simulink model "Cart_pole_adaptive_simulation"  (R2025b)
settings: Solver=ode4  StartTime=0.0  StopTime=10  FixedStep=0.025  RelTol=1e-3
values from neighbouring files (symbols this model uses):
  m = 0.7    [cart_pole_model.m]    (also in cart_pole_model_2.m = SX.sym('m'))
  N = 10    [cart_pole_mhe.m]    (also in cart_pole_ocp.m = 40; test.m = round(T_sim/dt))
  s = sin(theta)    [cart_pole_adaptive_model.m]    (also in cart_pole_model.m; cart_pole_model_2.m; test.m = sin(th))
  T = 1    [cart_pole_ocp.m]
undefined symbols (not defined in the file or in its folder): X, Y, Z
libraries: sm_lib x14, nesl_utility x7
settings Model: Creator=oj  LastModifiedBy=angel
settings SolverCC: AlgebraicLoopSolver=TrustRegion
settings DataIOCC: SaveFormat=StructureWithTime
settings OptimizationCC: LifeSpan=inf
settings DebuggingCC: UnconnectedInputMsg=warning  UnconnectedOutputMsg=warning  UnconnectedLineMsg=warning  SFExecutionAtInitializationDiag=none  ArithmeticOperatorsInVariantConditions=warning
settings HardwareCC: ProdBitPerSizeT=32.0  ProdBitPerPtrDiffT=32.0  ProdWordSize=32.0  ProdHWDeviceType=Specified
settings ModelReferenceCC: EnableRefExpFcnMdlSchedulingChecks=on
settings SFSimCC: CustomCodeUndefinedFunction=UseInterfaceOnly
settings RTWCC: GPUComputeCapability=3.5
settings CodeAppCC: StateflowObjectComments=on
settings ExplorerConfigSet: InternalSimMechanicsExplorerSettings=|
  | <ExplorerConfiguration>
  | 
  |   <canonicalview>default</canonicalview>
  | 
  |   <TilePanel>
  |     <TileInfo>
  |       <Tiles Columns="1" Count="1" Height="858" Rows="1" Width="1140">
  |         <Row Weight="1"/>
  |         <Column Weight="1"/>
  |         <Tile Height="1" Width="1" X="0" Y="0"/>
  |       </Tiles>
  |     </TileInfo>
  |     <SceneInfo>
  |       <SceneViewer>
  |         <IsThisViewStd>
  |           <IsStandardView>off</IsStandardView>
  |           <StandardViewName>Front</StandardViewName>
  |         </IsThisViewStd>
  |         <BGColor>
  |           <R>1</R>
  |           <G>1</G>
  |           <B>1</B>
  |           <A>1</A>
  |         </BGColor>
  |         <Camera>
  |           <DoPerspective>off</DoPerspective>
  |           <Position>
  |             <X>0.79287567589367203</X>
  |             <Y>-2.8977650595772118</Y>
  |             <Z>0.43288588007438944</Z>
  |           </Position>
  |           <Center>
  |             <X>0.09273481289714941</X>
  |             <Y>-0.01114024585481534</Y>
  |             <Z>-0.08401232882620252</Z>
  |           </Center>
  |           <Up>
  |             <X>-0.027084665030150518</X>
  |             <Y>0.16982947078524466</Y>
  |             <Z>0.98510119874711777</Z>
  |           </Up>
  |           <XLim>0.48380424524844262</XLim>
  |           <YLim>0.48380424524844262</YLim>
  |           <ViewLimDist>0.01</ViewLimDist>
  |         </Camera>
  |       </SceneViewer>
  |     </SceneInfo>
  |   </TilePanel>
  | 
  |   <MechEditorPanel>
  |     <GfxPanelCameraMap/>
  |     <Cameras/>
  |     <VideoCreator>
  |       <IncludeTiles>All</IncludeTiles>
  |       <IncludeTime>on</IncludeTime>
  |       <IncludeWorldFrame>off</IncludeWorldFrame>
  |       <PlaybackSpeedRatio>1</PlaybackSpeedRatio>
  |       <FrameRate>30</FrameRate>
  |       <FrameSize>auto</FrameSize>
  |       <VideoFormat>UncompressedAVI</VideoFormat>
  |     </VideoCreator>
  |   </MechEditorPanel>
  | 
  |   <PlaybackSettings>
  |     <PlaybackSpeedFactor>1</PlaybackSpeedFactor>
  |   </PlaybackSettings>
  | 
  | </ExplorerConfiguration>

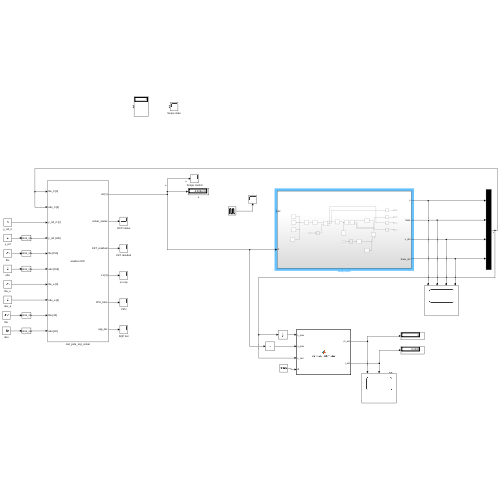
[thumbnail: Simulink's stored preview of the top-level diagram]
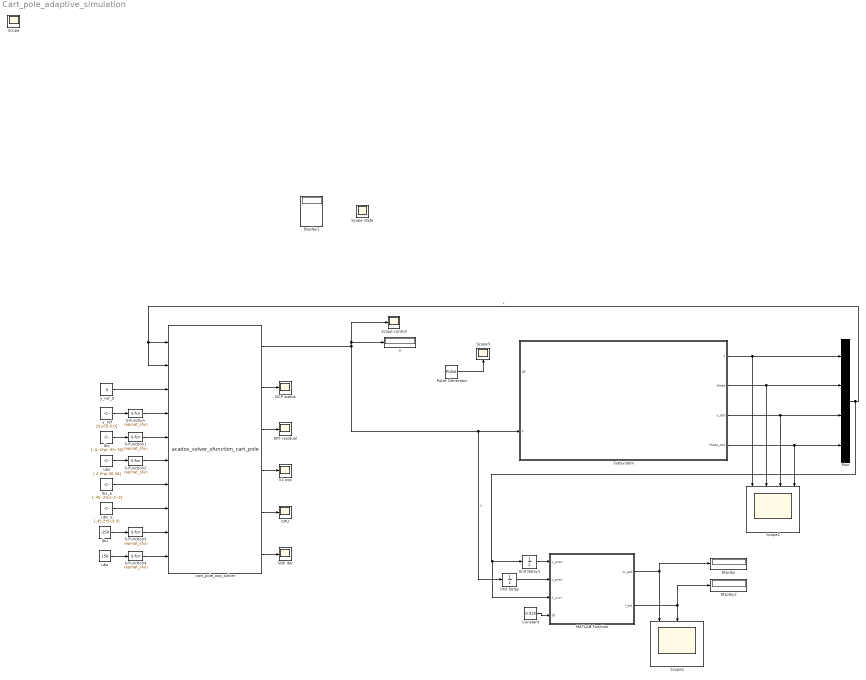
== system Cart_pole_adaptive_simulation ==
  CPU : Scope
      settings: Description=status  DataLoggingVariableName=ScopeData3
  Constant : Constant  Value=0.025
  Display : Display
  Display1 : Display
  Display2 : Display
  KKT residual : Scope
      settings: Description=status  ActiveDisplayYMinimum=-3E-6  ActiveDisplayYMaximum=3.1E-5  DataLoggingVariableName=ScopeData4
  MATLAB Function : MATLAB Function  TreatAsAtomicUnit=on
  Mux : Mux
  OCP status : Scope
      settings: Description=status  ActiveDisplayYMinimum=-4.610104567980212  ActiveDisplayYMaximum=5.6802344204737647
  Pulse Generator : DiscretePulseGenerator  PulseType=Time based  Period=10  PulseWidth=10  PhaseDelay=3
  S-Function : S-Function  FunctionName=repmat_sfun  Parameters=N/T-1  SFunctionDeploymentMode=off  EnableBusSupport=off
  S-Function1 : S-Function  FunctionName=repmat_sfun  Parameters=N/T-1  SFunctionDeploymentMode=off  EnableBusSupport=off
  S-Function2 : S-Function  FunctionName=repmat_sfun  Parameters=N/T-1  SFunctionDeploymentMode=off  EnableBusSupport=off
  S-Function3 : S-Function  FunctionName=repmat_sfun  Parameters=N  SFunctionDeploymentMode=off  EnableBusSupport=off
  S-Function4 : S-Function  FunctionName=repmat_sfun  Parameters=N  SFunctionDeploymentMode=off  EnableBusSupport=off
  SQP iter : Scope
      settings: Description=status  DataLoggingVariableName=ScopeData5
  Scope control : Scope
      settings: ActiveDisplayYMinimum=383.73133875981432  ActiveDisplayYMaximum=527.06243125068556  DataLoggingVariableName=ScopeData6
  Scope state : Scope
      settings: ActiveDisplayYMinimum=-11.71868  ActiveDisplayYMaximum=10.42658  DataLoggingVariableName=ScopeData7
  Scope1 : Scope  NumInputPorts=4
      settings: ActiveDisplayYMinimum=-6.4000749439613926  ActiveDisplayYMaximum=35.778508565711434  DataLoggingVariableName=ScopeData8
  Scope2 : Scope  NumInputPorts=3
      settings: ActiveDisplayYMinimum=-0.18546513291642433  ActiveDisplayYMaximum=1.4995284530805071  DataLoggingVariableName=ScopeData9
  Scope3 : Scope
      settings: ActiveDisplayYMinimum=-1  ActiveDisplayYMaximum=1  DataLoggingVariableName=ScopeData10
  Subsystem : Subsystem
  Unit Delay : UnitDelay  SampleTime=-1  HasFrameUpgradeWarning=on
  Unit Delay1 : UnitDelay  SampleTime=-1  HasFrameUpgradeWarning=on
  cart_pole_ocp_solver : S-Function  FunctionName=acados_solver_sfunction_cart_pole  SFunctionDeploymentMode=off  EnableBusSupport=off
      mask Display:
      | global sfun_input_names sfun_output_names
      | for i = 1:length(sfun_input_names)
      |     port_label('input', i, sfun_input_names{i})
      | end
      | for i = 1:length(sfun_output_names)
      |     port_label('output', i, sfun_output_names{i})
      | end
      | disp("acados OCP")
  lbu : Constant  Value=-150
  lbx : Constant  Value=[-.4;-2*pi;-30;-30]
  lbx_e : Constant  Value=[-.45;-2*pi;-3;-3]
  u : Display
  ubu : Constant  Value=150
  ubx : Constant  Value=[.4;2*pi;30;30]
  ubx_e : Constant  Value=[.45;2*pi;3;3]
  x1 ocp : Scope
      settings: Description=status  ActiveDisplayYMinimum=-2E-10  ActiveDisplayYMaximum=2.6E-9  DataLoggingVariableName=ScopeData2
  y_ref : Constant  Value=[0;pi;0;0;0]
  y_ref_0 : Constant  Value=0
  Scope : Scope
      settings: ActiveDisplayYMinimum=-13.79726  ActiveDisplayYMaximum=10.28583
  wires:
  lbu/1 -> S-Function3/1
  cart_pole_ocp_solver/1 -> Scope control/1, u/1, Unit Delay/1, Subsystem/2(F)  "u"
  y_ref/1 -> S-Function/1
  lbx_e/1 -> cart_pole_ocp_solver/7
  cart_pole_ocp_solver/5 -> CPU/1
  cart_pole_ocp_solver/6 -> SQP iter/1
  cart_pole_ocp_solver/3 -> KKT residual/1
  ubx_e/1 -> cart_pole_ocp_solver/8
  ubx/1 -> S-Function2/1
  lbx/1 -> S-Function1/1
  cart_pole_ocp_solver/4 -> x1 ocp/1
  cart_pole_ocp_solver/2 -> OCP status/1
  y_ref_0/1 -> cart_pole_ocp_solver/3
  Subsystem/1(x) -> Mux/1, Scope1/1
  Subsystem/3(x_dot) -> Mux/3, Scope1/3
  Subsystem/4(theta_dot) -> Mux/4, Scope1/4
  Subsystem/2(theta) -> Mux/2, Scope1/2
  S-Function/1 -> cart_pole_ocp_solver/4
  Mux/1 -> MATLAB Function/3(x_curr), Unit Delay1/1, cart_pole_ocp_solver/2, cart_pole_ocp_solver/1  "x"
  Pulse Generator/1 -> Scope3/1
  S-Function1/1 -> cart_pole_ocp_solver/5
  S-Function2/1 -> cart_pole_ocp_solver/6
  S-Function3/1 -> cart_pole_ocp_solver/9
  S-Function4/1 -> cart_pole_ocp_solver/10
  ubu/1 -> S-Function4/1
  MATLAB Function/1(m_est) -> Display/1, Scope2/1
  MATLAB Function/2(I_est) -> Display2/1, Scope2/2
  Constant/1 -> MATLAB Function/4(dt)
  Unit Delay/1 -> MATLAB Function/2(u_prev)
  Unit Delay1/1 -> MATLAB Function/1(x_prev)

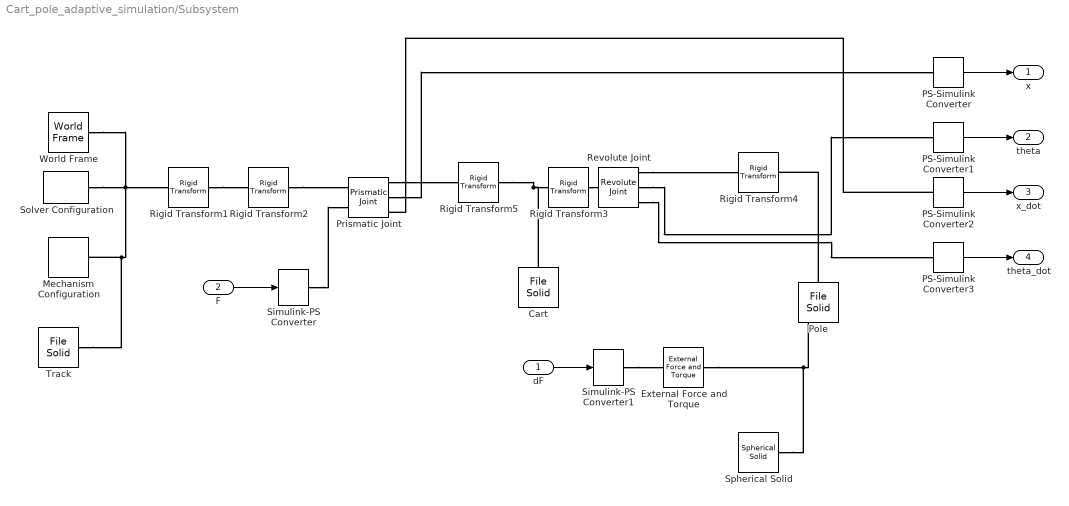
== system Cart_pole_adaptive_simulation/Subsystem ==
  dF : Inport
  F : Inport  Port=2
  Cart : sm_lib/Body Elements/File Solid  ExtGeomFileName=/home/angel/Projects/master-thesis/Projects/cart_pole/STEP/Cart.stp  UnitType=FromFile  ExtGeomFileUnits=m  StepReaderType=HEX  ExportConvexHullGeometry=off  InertiaType=CalculateFromGeometry  BasedOnType=Density  Density=density_steel  DensityUnits=kg/m^3  Mass=1  MassUnits=kg  CenterOfMass=[0 0 0]  CenterOfMassUnits=m  MomentsOfInertia=[1 1 1]  MomentsOfInertiaUnits=kg*m^2  ProductsOfInertia=[0 0 0]  ProductsOfInertiaUnits=kg*m^2  GraphicType=FromGeometry  MarkerShape=Sphere  MarkerSize=10  GraphicVisPropType=SimpleVisualProperties  GraphicDiffuseColor=[0.502 0.1059 0.1059]  GraphicOpacity=1  GraphicSpecularColor=[0.5 0.5 0.5 1.0]  GraphicAmbientColor=[0.15 0.15 0.15 1.0]  GraphicEmissiveColor=[0.0 0.0 0.0 1.0]  GraphicShininess=75  DoExposeReferenceFrame=on  SerializedFrames=<Frames/>
  External Force and Torque : sm_lib/Forces and Torques/External Force and Torque  EnableForceX=on  EnableForceY=off  EnableForceZ=off  EnableForce=off  ForceResolutionFrame=World  EnableTorqueX=off  EnableTorqueY=off  EnableTorqueZ=off  EnableTorque=off  TorqueResolutionFrame=AttachedFrame
  Mechanism Configuration : sm_lib/Utilities/Mechanism Configuration  UniformGravity=Constant  GravityVector=[0 0 -9.81]  GravityVectorUnits=m/s^2  LinearizationDelta=0.001  JointModeTransitionNonlinearIterations=2
  PS-Simulink Converter{,1..3} (4 alike) : nesl_utility/PS-Simulink Converter  PhysicalDomain=network_engine_domain  SubClassName=ps_output  LeftPortType=input  RightPortType=output  PseudoPeriodic=off  Frequencies=[]  VectorFormat=1-D array  Unit=1  AffineConversion=off
  Pole : sm_lib/Body Elements/File Solid  ExtGeomFileName=/home/angel/Projects/master-thesis/Projects/cart_pole/STEP/Pole.stp  UnitType=FromFile  ExtGeomFileUnits=m  StepReaderType=HEX  ExportConvexHullGeometry=on  InertiaType=CalculateFromGeometry  BasedOnType=Density  Density=density_steel  DensityUnits=kg/m^3  Mass=1  MassUnits=kg  CenterOfMass=[0 0 0]  CenterOfMassUnits=m  MomentsOfInertia=[1 1 1]  MomentsOfInertiaUnits=kg*m^2  ProductsOfInertia=[0 0 0]  ProductsOfInertiaUnits=kg*m^2  GraphicType=FromGeometry  MarkerShape=Sphere  MarkerSize=10  GraphicVisPropType=SimpleVisualProperties  GraphicDiffuseColor=[0.5843 0.5843 0.5843]  GraphicOpacity=1  GraphicSpecularColor=[0.5 0.5 0.5 1.0]  GraphicAmbientColor=[0.15 0.15 0.15 1.0]  GraphicEmissiveColor=[0.0 0.0 0.0 1.0]  GraphicShininess=75  DoExposeReferenceFrame=on  SerializedFrames=|
      | <Frames>
      | 
      |   <Frame>
      |     <Id>Frame1</Id>
      |     <Value>
      |       <Name>S</Name>
      |       <Origin>
      |         <Source>GeometricFeature</Source>
      |         <FeatureName>spherical surface 2</FeatureName>
      |       </Origin>
      |       <PrimaryAxis>
      |         <DefinedDirection>+Z</DefinedDirection>
      |         <Source>ReferenceFrame</Source>
      |         <SourceDirection>+Z</SourceDirection>
      |         <FeatureName></FeatureName>
      |       </PrimaryAxis>
      |       <SecondaryAxis>
      |         <DefinedDirection>+X</DefinedDirection>
      |         <Source>ReferenceFrame</Source>
      |         <SourceDirection>+X</SourceDirection>
      |         <FeatureName></FeatureName>
      |       </SecondaryAxis>
      |     </Value>
      |   </Frame>
      | 
      | </Frames>
  Prismatic Joint : sm_lib/Joints/Prismatic Joint  JointMode=Normal  CompositeWrenchDir=FollowerOnBase  CompositeWrenchFrame=BaseFrame  SenseConstraintForce=off  SenseConstraintTorque=off  SenseTotalForce=off  SenseTotalTorque=off  PositionTargetSpecify=off  PositionTargetPriority=High  PositionTargetValue=0  PositionTargetValueUnits=m  VelocityTargetSpecify=off  VelocityTargetPriority=High  VelocityTargetValue=0  VelocityTargetValueUnits=m/s  EquilibriumPosition=0  EquilibriumPositionUnits=m  SpringStiffness=0  SpringStiffnessUnits=N/m  DampingCoefficient=0  DampingCoefficientUnits=N/(m/s)  LowerLimitSpecify=off  LowerLimitBound=-.45  LowerLimitBoundUnits=m  LowerLimitStiffness=1e6  LowerLimitStiffnessUnits=N/m  LowerLimitDamping=1e3  LowerLimitDampingUnits=N/(m/s)  LowerLimitTransitionRegionWidth=1e-4  LowerLimitTransitionRegionWidthUnits=m  UpperLimitSpecify=off  UpperLimitBound=.45  UpperLimitBoundUnits=m  UpperLimitStiffness=1e6  UpperLimitStiffnessUnits=N/m  UpperLimitDamping=1e3  UpperLimitDampingUnits=N/(m/s)  UpperLimitTransitionRegionWidth=1e-4  UpperLimitTransitionRegionWidthUnits=m  TorqueActuationMode=InputTorque  MotionActuationMode=ComputedMotion  SensePosition=on  SenseVelocity=on  SenseAcceleration=off  SenseTorqueForce=off  SenseLowerLimitTorqueForce=off  SenseUpperLimitTorqueForce=off
  Revolute Joint : sm_lib/Joints/Revolute Joint  JointMode=Normal  CompositeWrenchDir=FollowerOnBase  CompositeWrenchFrame=BaseFrame  SenseConstraintForce=off  SenseConstraintTorque=off  SenseTotalForce=off  SenseTotalTorque=off  PositionTargetSpecify=on  PositionTargetPriority=High  PositionTargetValue=0  PositionTargetValueUnits=deg  VelocityTargetSpecify=off  VelocityTargetPriority=High  VelocityTargetValue=0  VelocityTargetValueUnits=deg/s  EquilibriumPosition=0  EquilibriumPositionUnits=deg  SpringStiffness=0  SpringStiffnessUnits=N*m/deg  DampingCoefficient=0  DampingCoefficientUnits=N*m/(rad/s)  LowerLimitSpecify=off  LowerLimitBound=-90  LowerLimitBoundUnits=deg  LowerLimitStiffness=1e4  LowerLimitStiffnessUnits=N*m/deg  LowerLimitDamping=10  LowerLimitDampingUnits=N*m/(deg/s)  LowerLimitTransitionRegionWidth=0.1  LowerLimitTransitionRegionWidthUnits=deg  UpperLimitSpecify=off  UpperLimitBound=90  UpperLimitBoundUnits=deg  UpperLimitStiffness=1e4  UpperLimitStiffnessUnits=N*m/deg  UpperLimitDamping=10  UpperLimitDampingUnits=N*m/(deg/s)  UpperLimitTransitionRegionWidth=0.1  UpperLimitTransitionRegionWidthUnits=deg  TorqueActuationMode=NoTorque  MotionActuationMode=ComputedMotion  SensePosition=on  SenseVelocity=on  SenseAcceleration=off  SenseTorqueForce=off  SenseLowerLimitTorqueForce=off  SenseUpperLimitTorqueForce=off
  Rigid Transform1 : sm_lib/Frames and Transforms/Rigid Transform  RotationMethod=StandardAxis  FollAlignAxisA=+X  BaseAlignAxisA=+Y  FollAlignAxisB=+Y  BaseAlignAxisB=+Z  RotationStandardAxis=+Y  RotationAngle=90  RotationAngleUnits=deg  RotationArbitraryAxis=[0 0 1]  RotationSequenceAxes=FollowerAxes  RotationSequence=XYX  RotationSequenceAngles=[0 0 0]  RotationSequenceAnglesUnits=deg  RotationMatrix=[1 0 0; 0 1 0; 0 0 1]  Quaternion=[1 0 0 0]  TranslationMethod=Cartesian  TranslationCartesianOffset=[0 0 0.1]  TranslationCartesianOffsetUnits=m  TranslationStandardAxis=+Z  TranslationStandardOffset=0  TranslationStandardOffsetUnits=m  TranslationROffset=0  TranslationROffsetUnits=m  TranslationThetaOffset=0  TranslationThetaOffsetUnits=deg  TranslationZOffset=0  TranslationZOffsetUnits=m
  Rigid Transform2 : sm_lib/Frames and Transforms/Rigid Transform  RotationMethod=StandardAxis  FollAlignAxisA=+X  BaseAlignAxisA=+Y  FollAlignAxisB=+Y  BaseAlignAxisB=+Z  RotationStandardAxis=+Z  RotationAngle=180  RotationAngleUnits=deg  RotationArbitraryAxis=[0 0 1]  RotationSequenceAxes=FollowerAxes  RotationSequence=XYX  RotationSequenceAngles=[0 0 0]  RotationSequenceAnglesUnits=deg  RotationMatrix=[1 0 0; 0 1 0; 0 0 1]  Quaternion=[1 0 0 0]  TranslationMethod=None  TranslationCartesianOffset=[0 0 0]  TranslationCartesianOffsetUnits=m  TranslationStandardAxis=+Z  TranslationStandardOffset=0  TranslationStandardOffsetUnits=m  TranslationROffset=0  TranslationROffsetUnits=m  TranslationThetaOffset=0  TranslationThetaOffsetUnits=deg  TranslationZOffset=0  TranslationZOffsetUnits=m
  Rigid Transform3 : sm_lib/Frames and Transforms/Rigid Transform  RotationMethod=StandardAxis  FollAlignAxisA=+X  BaseAlignAxisA=+Y  FollAlignAxisB=+Y  BaseAlignAxisB=+Z  RotationStandardAxis=-X  RotationAngle=90  RotationAngleUnits=deg  RotationArbitraryAxis=[0 0 1]  RotationSequenceAxes=FollowerAxes  RotationSequence=XYX  RotationSequenceAngles=[0 0 0]  RotationSequenceAnglesUnits=deg  RotationMatrix=[1 0 0; 0 1 0; 0 0 1]  Quaternion=[1 0 0 0]  TranslationMethod=Cartesian  TranslationCartesianOffset=[0 0 200]  TranslationCartesianOffsetUnits=mm  TranslationStandardAxis=+Z  TranslationStandardOffset=0  TranslationStandardOffsetUnits=m  TranslationROffset=0  TranslationROffsetUnits=m  TranslationThetaOffset=0  TranslationThetaOffsetUnits=deg  TranslationZOffset=0  TranslationZOffsetUnits=m
  Rigid Transform4 : sm_lib/Frames and Transforms/Rigid Transform  RotationMethod=StandardAxis  FollAlignAxisA=+X  BaseAlignAxisA=+Y  FollAlignAxisB=+Y  BaseAlignAxisB=+Z  RotationStandardAxis=-X  RotationAngle=90  RotationAngleUnits=deg  RotationArbitraryAxis=[0 0 1]  RotationSequenceAxes=FollowerAxes  RotationSequence=XYX  RotationSequenceAngles=[0 0 0]  RotationSequenceAnglesUnits=deg  RotationMatrix=[1 0 0; 0 1 0; 0 0 1]  Quaternion=[1 0 0 0]  TranslationMethod=Cartesian  TranslationCartesianOffset=[0 -200 0]  TranslationCartesianOffsetUnits=mm  TranslationStandardAxis=+X  TranslationStandardOffset=-0.025  TranslationStandardOffsetUnits=m  TranslationROffset=0  TranslationROffsetUnits=m  TranslationThetaOffset=0  TranslationThetaOffsetUnits=deg  TranslationZOffset=0  TranslationZOffsetUnits=m
  Rigid Transform5 : sm_lib/Frames and Transforms/Rigid Transform  RotationMethod=StandardAxis  FollAlignAxisA=+X  BaseAlignAxisA=+Y  FollAlignAxisB=+Y  BaseAlignAxisB=+Z  RotationStandardAxis=+Y  RotationAngle=90  RotationAngleUnits=deg  RotationArbitraryAxis=[0 0 1]  RotationSequenceAxes=FollowerAxes  RotationSequence=XYX  RotationSequenceAngles=[0 0 0]  RotationSequenceAnglesUnits=deg  RotationMatrix=[1 0 0; 0 1 0; 0 0 1]  Quaternion=[1 0 0 0]  TranslationMethod=Cartesian  TranslationCartesianOffset=[-0.1 0 0]  TranslationCartesianOffsetUnits=m  TranslationStandardAxis=+Z  TranslationStandardOffset=0  TranslationStandardOffsetUnits=m  TranslationROffset=0  TranslationROffsetUnits=m  TranslationThetaOffset=0  TranslationThetaOffsetUnits=deg  TranslationZOffset=0  TranslationZOffsetUnits=m
  Simulink-PS Converter : nesl_utility/Simulink-PS Converter  PhysicalDomain=network_engine_domain  SubClassName=ps_input  LeftPortType=input  RightPortType=output  PseudoPeriodic=off  Frequencies=[]  NoiseDistribution=none  NoiseParameters=[]  Unit=1  AffineConversion=off  FilteringAndDerivatives=zero  SimscapeFilterOrder=1  InputFilterTimeConstant=0.001  UdotUserProvided=1
  Simulink-PS Converter1 : nesl_utility/Simulink-PS Converter  PhysicalDomain=network_engine_domain  SubClassName=ps_input  LeftPortType=input  RightPortType=output  PseudoPeriodic=off  Frequencies=[]  NoiseDistribution=none  NoiseParameters=[]  Unit=1  AffineConversion=off  FilteringAndDerivatives=zero  SimscapeFilterOrder=1  InputFilterTimeConstant=0.001  UdotUserProvided=1
  Solver Configuration : nesl_utility/Solver Configuration  PhysicalDomain=network_engine_domain  SubClassName=solver  LeftPortType=input  RightPortType=generic  Tones=[]  Harmonics=[]  SimulateNoise=off  Profile=off  UseLocalSampling=off  EnableSwitchedLinearOptims=on  FrequencyDomain=off  UseCCode=off  RelTol=0.001  AbsTol=1e-06  MinStep=1e-09  ToWorkspace=off  RevertToSquareIcSolve=off  NumHomotopyIterations=100  PhasorMode=off  PhasorModeNumHarmonics=1  ConsistencySolver=NEWTON_FTOL  IndexReductionMethod=DerivativeReplacement  DoDC=off  ResidualTolerance=1e-09  ConsistencyTolSource=GLOBAL  ConsistencyAbsTol=0.001  ConsistencyRelTol=0.001  ConsistencyTolFactor=0.001  UseLocalSolver=off  LocalSolverChoice=NE_BACKWARD_EULER_ADVANCER  ResolveIndetEquations=on  FunctionEvalNumThread=1  LocalSolverSampleTime=0.001  DoFixedCost=off  MaxNonlinIter=3  MaxModeIter=2  ComputeImpulses=off  ImpulseIterations=2  LinearAlgebra=Sparse  LinearAlgebraNumThread=0  EquationFormulation=NE_TIME_EF  DelaysMemoryBudget=1024  AutomaticFiltering=on  FilteringTimeConstant=0.001  PartitionStorageMethod=AS_NEEDED  PartitionMemoryBudget=1024  PartitionMethod=FAST  MultibodyUseLocalSolver=off  MultibodyLocalSolverChoice=ODE1  MultibodyLocalSolverSampleTime=0.001
  Spherical Solid : sm_lib/Body Elements/Spherical Solid  SphereRadius=30  SphereRadiusUnits=mm  ExportEntireGeometry=off  InertiaType=CalculateFromGeometry  BasedOnType=Mass  Density=1000  DensityUnits=kg/m^3  Mass=0.4  MassUnits=kg  CenterOfMass=[0 0 0]  CenterOfMassUnits=m  MomentsOfInertia=[1 1 1]  MomentsOfInertiaUnits=kg*m^2  ProductsOfInertia=[0 0 0]  ProductsOfInertiaUnits=kg*m^2  GraphicType=FromGeometry  MarkerShape=Sphere  MarkerSize=10  GraphicVisPropType=SimpleVisualProperties  GraphicDiffuseColor=[0.7608 0.6706 0.3176]  GraphicOpacity=1  GraphicSpecularColor=[0.5 0.5 0.5 1.0]  GraphicAmbientColor=[0.15 0.15 0.15 1.0]  GraphicEmissiveColor=[0.0 0.0 0.0 1.0]  GraphicShininess=75  DoExposeReferenceFrame=on  SerializedFrames=<Frames/>
  Track : sm_lib/Body Elements/File Solid  ExtGeomFileName=/home/angel/Projects/master-thesis/Projects/cart_pole/STEP/Track.stp  UnitType=FromFile  ExtGeomFileUnits=m  StepReaderType=HEX  ExportConvexHullGeometry=off  InertiaType=CalculateFromGeometry  BasedOnType=Density  Density=1  DensityUnits=kg/m^3  Mass=1  MassUnits=kg  CenterOfMass=[0 0 0]  CenterOfMassUnits=m  MomentsOfInertia=[1 1 1]  MomentsOfInertiaUnits=kg*m^2  ProductsOfInertia=[0 0 0]  ProductsOfInertiaUnits=kg*m^2  GraphicType=FromGeometry  MarkerShape=Sphere  MarkerSize=10  GraphicVisPropType=SimpleVisualProperties  GraphicDiffuseColor=[0.5 0.5 0.5]  GraphicOpacity=1  GraphicSpecularColor=[0.5 0.5 0.5 1.0]  GraphicAmbientColor=[0.15 0.15 0.15 1.0]  GraphicEmissiveColor=[0.0 0.0 0.0 1.0]  GraphicShininess=75  DoExposeReferenceFrame=on  SerializedFrames=<Frames/>
  World Frame : sm_lib/Frames and Transforms/World Frame
  x : Outport  VectorParamsAs1DForOutWhenUnconnected=off
  theta : Outport  Port=2  VectorParamsAs1DForOutWhenUnconnected=off
  x_dot : Outport  Port=3  VectorParamsAs1DForOutWhenUnconnected=off
  theta_dot : Outport  Port=4  VectorParamsAs1DForOutWhenUnconnected=off
  wires:
  PS-Simulink Converter1/1 -> theta/1
  dF/1 -> Simulink-PS Converter1/1
  PS-Simulink Converter/1 -> x/1
  PS-Simulink Converter3/1 -> theta_dot/1
  PS-Simulink Converter2/1 -> x_dot/1
  F/1 -> Simulink-PS Converter/1
  connections:
  Rigid Transform2/RConn1 -- Prismatic Joint/LConn1
  Prismatic Joint/RConn2 -- PS-Simulink Converter/LConn1
  Rigid Transform3/RConn1 -- Revolute Joint/LConn1
  Revolute Joint/RConn3 -- PS-Simulink Converter3/LConn1
  Simulink-PS Converter1/RConn1 -- External Force and Torque/LConn1
  Simulink-PS Converter/RConn1 -- Prismatic Joint/LConn2
  Pole/RConn1 -- Rigid Transform4/RConn1
  World Frame/RConn1 -- Rigid Transform1/LConn1 -- Track/RConn1 -- Mechanism Configuration/RConn1 -- Solver Configuration/RConn1
  Revolute Joint/RConn1 -- Rigid Transform4/LConn1
  PS-Simulink Converter2/LConn1 -- Prismatic Joint/RConn3
  Prismatic Joint/RConn1 -- Rigid Transform5/LConn1
  Rigid Transform1/RConn1 -- Rigid Transform2/LConn1
  Revolute Joint/RConn2 -- PS-Simulink Converter1/LConn1
  Rigid Transform5/RConn1 -- Cart/RConn1 -- Rigid Transform3/LConn1
  External Force and Torque/RConn1 -- Spherical Solid/RConn1 -- Pole/LConn1

== matlab function Cart_pole_adaptive_simulation/MATLAB Function ==
  settings: updateMethod=DISCRETE
  data: x_prev input; m_est output; u_prev input; x_curr input; dt input; I_est output
function [m_est, I_est] = rls_mass_estimator(x_prev, u_prev, x_curr, dt)
% RLS para estimar masa del péndulo en Simulink
%   x_prev: estado en paso anterior [p; theta; v; omega] (4x1)
%   u_prev: control aplicado en paso anterior (1x1)
%   x_curr: estado medido actual (4x1)
%   dt:    paso de tiempo de simulación (1x1)
%
%   Salidas:
%   m_est: masa estimada del péndulo [kg]
%   I_est: inercia estimada [kg*m^2]

    % --- Variables persistentes (estado del estimador) ---
    persistent theta_hat P initialized
    
    % Inicialización primera vez
    if isempty(initialized)
        theta_hat = [0.3; 1e-4];      % [m; I] inicial arbitrario (erróneo)
        P = 1e4 * eye(2);             % covarianza inicial alta
        initialized = true;
    end
    
    % Parámetros físicos conocidos (carro + geometría)
    M = 7.67;    % masa carro [kg]
    L = 0.155;   % longitud péndulo [m]
    g = 9.81;    % gravedad [m/s^2]
    lambda = 0.995;  % factor de olvido
    
    % --- Solo actualizar si tenemos datos válidos (evitar t=0) ---
    if ~isempty(x_prev) && ~isempty(u_prev) && ~isempty(x_curr)
        % 1. Predicción con modelo usando parámetros actuales
        m_cur = theta_hat(1);
        I_cur = theta_hat(2);
        x_pred = predict_state(x_prev, u_prev, M, m_cur, L, I_cur, g, dt);
        
        % 2. Error de predicción (solo ángulo y velocidad angular)
        e = x_curr([2; 4]) - x_pred([2; 4]);
        
        % 3. Gradiente numérico ∂f/∂[m; I]
        eps_m = 1e-4;
        eps_I = 1e-6;
        
        x_m_pert = predict_state(x_prev, u_prev, M, m_cur+eps_m, L, I_cur, g, dt);
        df_dm = (x_m_pert([2;4]) - x_pred([2;4])) / eps_m;
        
        x_I_pert = predict_state(x_prev, u_prev, M, m_cur, L, I_cur+eps_I, g, dt);
        df_dI = (x_I_pert([2;4]) - x_pred([2;4])) / eps_I;
        
        phi = [df_dm, df_dI];  % matriz 2x2
        
        % 4. Actualización RLS
        denom = lambda + phi * P * phi';
        if abs(denom) > 1e-12
            K = (P * phi') / denom;
            theta_hat = theta_hat + K * e;
            P = (P - K * phi * P) / lambda;
        end
        
        % 5. Clamp físico (evitar valores no realistas)
        theta_hat(1) = max(0.1, min(5.0, theta_hat(1)));  % masa entre 0.1-5 kg
        I_min = 0.1 * theta_hat(1) * L^2;
        I_max = 2.0 * theta_hat(1) * L^2;
        theta_hat(2) = max(I_min, min(I_max, theta_hat(2)));
    end
    
    % Salidas
    m_est = theta_hat(1);
    I_est = theta_hat(2);
end

function x_next = predict_state(x, u, M, m, L, I, g, dt)
    % Predice siguiente estado con Euler explícito
    p = x(1); theta = x(2); v = x(3); omega = x(4);
    F = u;
    
    s = sin(theta);
    c = cos(theta);
    
    % Matriz de masa
    M11 = M + m;
    M12 = m * L * c;
    M22 = m * L^2 + I;
    M_mat = [M11, M12; M12, M22];
    
    % Vector de fuerzas
    rhs1 = F + m * L * s * omega^2;
    rhs2 = -m * g * L * s;
    rhs = [rhs1; rhs2];
    
    % Aceleraciones
    accel = M_mat \ rhs;
    a = accel(1);
    alpha = accel(2);
    
    % Integración Euler
    p_next = p + dt * v;
    theta_next = theta + dt * omega;
    v_next = v + dt * a;
    omega_next = omega + dt * alpha;
    
    x_next = [p_next; theta_next; v_next; omega_next];
end
